simulink model "vanderPol"  (R2024b)
settings: Solver=FixedStepAuto  StartTime=0.0  StopTime=100000  FixedStep=0.01  RelTol=1e-3
settings Model: Creator=castl  LastModifiedBy=castl

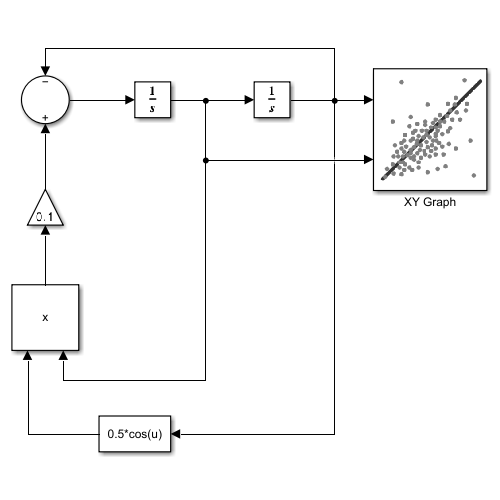
[thumbnail: Simulink's stored preview of the top-level diagram]
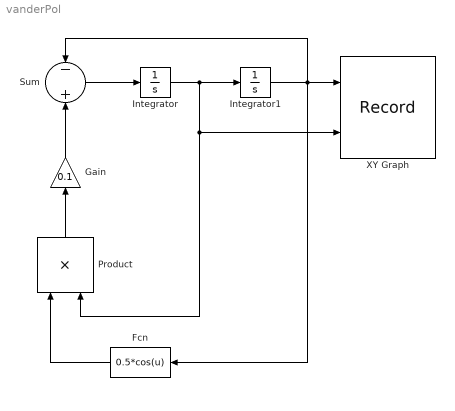
== system vanderPol ==
  Fcn : Fcn  Expr=0.5*cos(u)
  Gain : Gain  Gain=0.1
  Integrator : Integrator  InitialCondition=2
  Integrator1 : Integrator
  Product : Product
  Sum : Sum  Inputs=-+
  XY Graph : Record  FileSettingsInternal="{\"entries\":[{\"content\":{\"excelSettings\":{\"content\":{},\"type\":\"Streamout.ExcelSettings\"}},\"type\":\"Streamout.FileSettingStorage\",\"uuid\":\"\"}],\"packageUris\":[\"http:\\/\\/schema.mathworks.com\\/mf0\\/streamout_blocks\\/R2020a\"],\"version\":\"1.0\"}"  Layout=[1 1]  SignalsInternal="{\"entries\":[{\"content\":{\"signals\":[{\"content\":{\"blockPath\":[],\"dimensions\":[1],\"domain\":\"\",\"lineColor\":\"#a2142f\",\"plots\":[ 1 ],\"port\":1,\"sid\":[\"\"],\"signalID\":1,\"signalName\":\"Integrator1\"},\"type\":\"RecordBlkView.Signal\",\"uuid\":\"\"},{\"content\":{\"blockPath\":[],\"dimensions\":[1],\"domain\":\"\",\"lineColor\":\"#139fff\",\"plots\":[ 1 ],\"port\":2,\"sid\":[\"\"],\"signalID\":2,\"signalName\":\"Integrator\"},\"type\":\"RecordBlkView.Signal\",\"uuid\":\"\"}]},\"type\":\"RecordBlkView.InputSignals\",\"uuid\":\"\"}],\"packageUris\":[\"http:\\/\\/schema.mathworks.com\\/mf0\\/streamout_blocks\\/R2020a\"],\"version\":\"1.0\"}"  VisualizationBindings="{\"xyplotplugin\":{\"info\":[{\"series\":[{\"bindingParametersList\":[{\"parameter\":\"X-Axis\",\"signalID\":1,\"signalName\":\"Integrator1\"},{\"parameter\":\"Y-Axis\",\"signalID\":2,\"signalName\":\"Integrator\"}],\"seriesID\":0}],\"subplotID\":1}]}}"  CompatibilityTag=XY
  wires:
  Sum/1 -> Integrator/1
  Integrator/1 -> Product/2, XY Graph/2, Integrator1/1
  Integrator1/1 -> Fcn/1, Sum/1, XY Graph/1
  Product/1 -> Gain/1
  Gain/1 -> Sum/2
  Fcn/1 -> Product/1
